simulink model "SawToothMandani"  (R2018b)
settings: Solver=VariableStepAuto  StartTime=0.0  StopTime=400  RelTol=1e-3
values from neighbouring files (symbols this model uses):
  s1 = values(i)    [testyboi.m]
  s2 = values(j)    [testyboi.m]
libraries: fuzblock x1
settings Model: Creator=soren  LastModifiedBy=soren

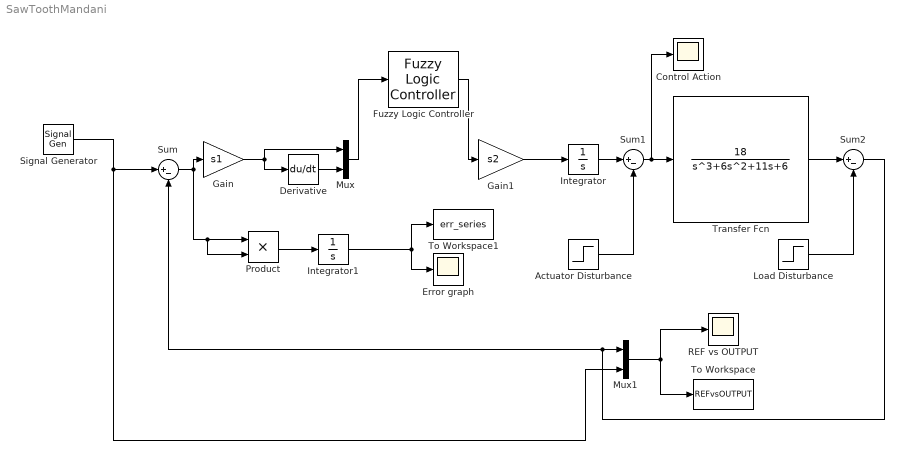
== system SawToothMandani ==
  "Actuator Disturbance " : Step  Time=200  SampleTime=0
  "Control Action " : Scope
  Derivative : Derivative
  "Error graph " : Scope
  Fuzzy Logic Controller : fuzblock/Fuzzy Logic  Controller  FIS=fis  OutputSampleNumber=101  DataType=double  FuzzifiedInputs=off  RuleFiringStrengths=off  RuleOutputs=off  AggregatedOutputs=off  SimulateUsing=Interpreted execution  OutOfRangeInputValueMessage=warning  NoRuleFiredMessage=warning  EmptyOutputFuzzySetMessage=warning
  Gain : Gain  Gain=s1  OutMin=-1  OutMax=1
  Gain1 : Gain  Gain=s2
  Integrator : Integrator
  Integrator1 : Integrator
  "Load Disturbance " : Step  Time=300  SampleTime=0
  Mux : Mux  Inputs=2
  Mux1 : Mux  Inputs=2
  Product : Product
  "REF vs OUTPUT " : Scope
  Signal Generator : SignalGenerator  WaveForm=sawtooth  Frequency=0.01
  Sum : Sum  Inputs=|+-
  Sum1 : Sum  Inputs=|+-
  Sum2 : Sum  Inputs=|+-
  To Workspace : ToWorkspace  VariableName=REFvsOUTPUT  SaveFormat=Timeseries  SampleTime=-1
  To Workspace1 : ToWorkspace  VariableName=err_series  SaveFormat=Timeseries  SampleTime=-1
  Transfer Fcn : TransferFcn  Numerator=[18]  Denominator=[1 6 11 6]
  wires:
  Signal Generator/1 -> Mux1/2, Sum/1
  Sum/1 -> Product/2, Product/1, Gain/1
  Gain/1 -> Mux/1, Derivative/1
  Derivative/1 -> Mux/2
  Mux/1 -> Fuzzy Logic Controller/1
  Fuzzy Logic Controller/1 -> Gain1/1
  Gain1/1 -> Integrator/1
  Integrator/1 -> Sum1/1
  Product/1 -> Integrator1/1
  Integrator1/1 -> To Workspace1/1, "Error graph "/1
  Mux1/1 -> To Workspace/1, "REF vs OUTPUT "/1
  Sum1/1 -> Transfer Fcn/1, "Control Action "/1
  Transfer Fcn/1 -> Sum2/1
  Sum2/1 -> Sum/2, Mux1/1
  "Actuator Disturbance "/1 -> Sum1/2
  "Load Disturbance "/1 -> Sum2/2
